simulink model "modello_motore_stato"  (R2014b)
settings: Solver=ode45  StartTime=0.0  StopTime=simulation_time  RelTol=1e-3
values from neighbouring files (symbols this model uses):
  A = [0, 1 ... (first row only)    [controllo_motore_modello_interno.m]    (also in controllo_motore_stato.m; controllo_motore_stato_integrale.m)
  B = [0 ... (first row only)    [controllo_motore_modello_interno.m]    (also in controllo_motore_stato.m; controllo_motore_stato_integrale.m)
  C = [c, 0]    [controllo_motore_modello_interno.m]    (also in controllo_motore_stato.m = [ c , 0]; controllo_motore_stato_integrale.m)
  d = 0    [controllo_motore_stato.m]    (also in controllo_motore_stato_integrale.m = -0.2; modello_motore.m = -0.5)
  K = acker (Az , Bz , W)    [controllo_motore_modello_interno.m]    (also in controllo_motore_stato.m = place ( A , B , W ); controllo_motore_stato_integrale.m = acker (Az, Bz, W))
  Kg2v = 5 / 176    (= 0.0284090909091)    [controllo_motore_modello_interno.m]    (also in controllo_motore_stato.m; controllo_motore_stato_integrale.m; modello_motore.m)
  N = 14    [controllo_motore_modello_interno.m]    (also in controllo_motore_stato.m = 11.8193119253; controllo_motore_stato_integrale.m; modello_motore.m)
  r = 50    [controllo_motore_stato.m]    (also in controllo_motore_stato_integrale.m = 120; modello_motore.m = 120)
settings Model: Creator=Nicola  LastModifiedBy=Nicola
settings SolverCC: AutoInsertRateTranBlk=on
settings DataIOCC: SaveOutput=off  SaveTime=off
settings OptimizationCC: InlineParams=on  InlineInvariantSignals=on  StateBitsets=on  DataBitsets=on  UseTempVars=on  ZeroExternalMemoryAtStartup=off  ZeroInternalMemoryAtStartup=off  NoFixptDivByZeroProtection=on  OptimizeModelRefInitCode=on  LifeSpan=1
settings DebuggingCC: UnderspecifiedInitializationDetection=Classic  MergeDetectMultiDrivingBlocksExec=none  StateNameClashWarn=warning
settings HardwareCC: ProdIntDivRoundTo=Floor  ProdEndianess=LittleEndian  ProdHWDeviceType=Generic->Custom
settings RTWCC: SystemTargetFile=ert.tlc  TLCOptions=-p0  GenCodeOnly=on  TemplateMakefile=ert_default_tmf  Description=Embedded Coder  GenerateReport=on  RTWVerbose=off  ProcessScript=ert_make_rtw_hook  IncludeHyperlinkInReport=on  LaunchReport=on
settings CodeAppCC: ForceParamTrailComments=on  IgnoreCustomStorageClasses=off  SimulinkDataObjDesc=on  CustomSymbolStrGlobalVar=rt$N$M  CustomSymbolStrType=$N$M  CustomSymbolStrFcn=$N$M$F  CustomSymbolStrMacro=$N$M  InsertBlockDesc=on
settings ERTTargetCC: TargetLangStandard=C99 (ISO)  GenerateSampleERTMain=on  IncludeMdlTerminateFcn=off  SuppressErrorStatus=on  SupportAbsoluteTime=off  SupportNonFinite=off  SupportComplex=off  PurelyIntegerCode=on  InlinedParameterPlacement=NonHierarchical  RootIOFormat=Structure reference  ERTCustomFileTemplate=example_file_process.tlc

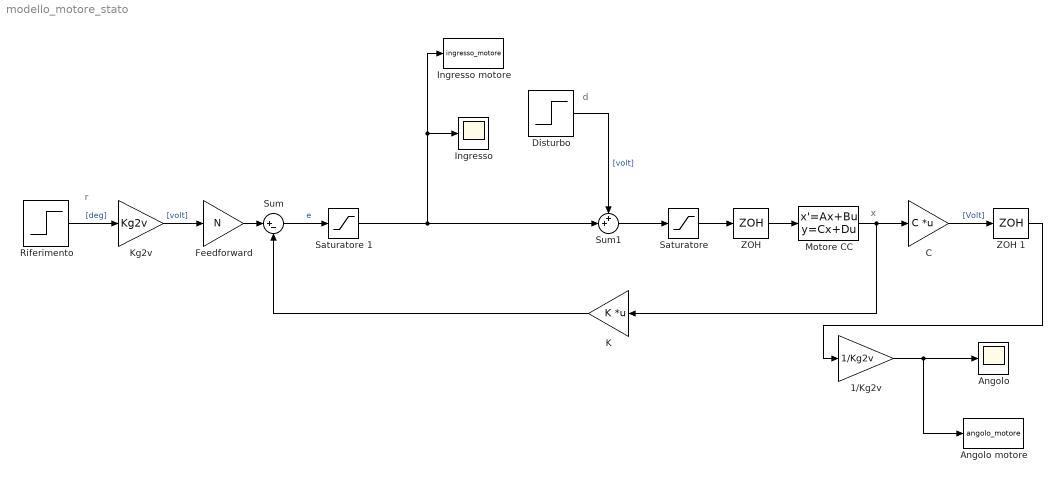
== system modello_motore_stato ==
  note: x
  note: d
  note: r
  "1/Kg2v " : Gain  Gain=1/Kg2v
  Angolo : Scope
  Angolo motore : ToWorkspace  VariableName=angolo_motore  SampleTime=-1
  C : Gain  Gain=C  Multiplication=Matrix(K*u)
  Disturbo : Step  After=d  SampleTime=0
  Feedforward : Gain  Gain=N
  Ingresso : Scope
  Ingresso motore : ToWorkspace  VariableName=ingresso_motore  SampleTime=-1
  K : Gain  Gain=K  Multiplication=Matrix(K*u)
  Kg2v : Gain  Gain=Kg2v
  Motore CC : StateSpace  A=A  B=B  C=eye(2)  D=[0; 0]  X0=0
  Riferimento : Step  After=r  SampleTime=0
  "Saturatore " : Saturate  UpperLimit=5  LowerLimit=-5
  Saturatore 1 : Saturate  UpperLimit=5  LowerLimit=-5
  Sum : Sum  Inputs=|+-
  Sum1 : Sum  Inputs=++|
  ZOH : ZeroOrderHold  SampleTime=0.001
  "ZOH 1 " : ZeroOrderHold  SampleTime=0.001
  wires:
  Riferimento/1 -> Kg2v/1  "[deg]"
  "Saturatore "/1 -> ZOH/1
  "1/Kg2v "/1 -> Angolo motore/1, Angolo/1
  Sum/1 -> Saturatore 1/1  "e"
  Saturatore 1/1 -> Sum1/2, Ingresso/1, Ingresso motore/1
  Sum1/1 -> "Saturatore "/1
  Disturbo/1 -> Sum1/1  "[volt]"
  Kg2v/1 -> Feedforward/1  "[volt]"
  Feedforward/1 -> Sum/1
  ZOH/1 -> Motore CC/1
  Motore CC/1 -> K/1, C/1
  C/1 -> "ZOH 1 "/1  "[Volt]"
  K/1 -> Sum/2
  "ZOH 1 "/1 -> "1/Kg2v "/1
